simulink model "full_3omni_ctrl_sim_and_exp_with_xpctarget"  (R2014b)
settings: Solver=ode3  SolverMode=SingleTasking  StartTime=0.0  StopTime=40  FixedStep=0.01  RelTol=1e-3
libraries: xpcobsoletelib x13, simulink x10, xpcutilitieslib x3, slrtlib x3
(part 1 of 2)
settings Model: SimulationMode=external  CovMetricSettings=dwe  CovHtmlReporting=off  covSaveCumulativeToWorkspaceVar=off  CovSaveSingleToWorkspaceVar=off  CovExternalEMLEnable=on  CovSFcnEnable=on  Creator=Sarot PC  LastModifiedBy=Sarot PC
settings DataIOCC: LimitDataPoints=off  SaveFormat=StructureWithTime  ReturnWorkspaceOutputs=on
settings OptimizationCC: BlockReduction=off  OptimizeBlockIOStorage=off  BufferReuse=off  GlobalBufferReuse=off  ExpressionFolding=off  LocalBlockOutputs=off
settings DebuggingCC: SolverPrmCheckMsg=none  FrameProcessingCompatibilityMsg=error  SFUnexpectedBacktrackingDiag=error  SFNoUnconditionalDefaultTransitionDiag=error
settings HardwareCC: ProdIntDivRoundTo=Zero  ProdEndianess=LittleEndian  ProdLongLongMode=on  ProdHWDeviceType=Generic->32-bit x86 compatible
settings ModelReferenceCC: PropagateSignalLabelsOutOfModel=on
settings SFSimCC: SimUseLocalCustomCode=on
settings RTWCC: Description=Simulink Real-Time  SystemTargetFile=slrt.tlc  TemplateMakefile=slrt_default_tmf  RTWUseLocalCustomCode=on  CodeExecutionProfiling=on  RTWCompilerOptimization=On
settings SimulinkRealTimeCC: GeneratePreprocessorConditionals=Disable all

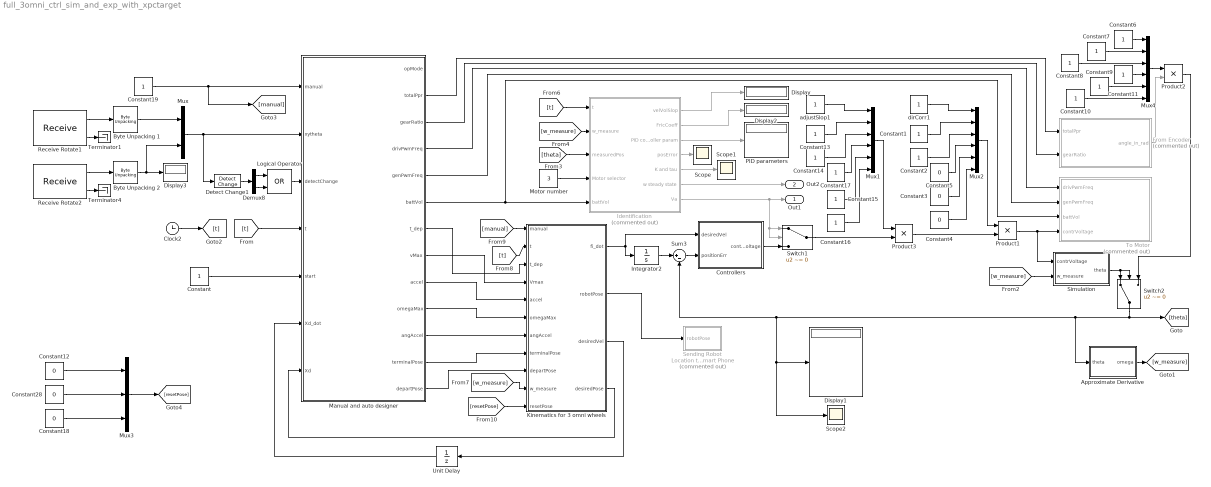
== system full_3omni_ctrl_sim_and_exp_with_xpctarget ==
  Approximate Derivative : Subsystem
  Byte Unpacking 1 : xpcutilitieslib/Byte Unpacking   MaskUnpackedDataTypes={'double'}  MaskUnpackedDataSizes={[1]}  MaskAlignment=1
  Byte Unpacking 2 : xpcutilitieslib/Byte Unpacking   MaskUnpackedDataTypes={'double'}  MaskUnpackedDataSizes={[1]}  MaskAlignment=1
  Clock2 : Clock
  Constant{,1..2,6..11,13..17,19} (15 alike) : Constant
  Constant{3..5,12,18,28} (6 alike) : Constant  Value=0
  Controllers : Subsystem
  Demux8 : Demux  Outputs=2
  Detect Change1 : simulink/Logic and Bit Operations/Detect Change  vinit=0  OutDataTypeStr=boolean
  Display{,1..3} (4 alike) : Display
  From Encoder : Subsystem  Commented=on
  Identification : Subsystem  Commented=on
  Integrator2 : Integrator  InitialCondition=zeros(6,1)
  Kinematics for 3 omni wheels : Subsystem
  Logical Operator : Logic  Operator=OR  AllPortsSameDT=off  OutDataTypeStr=boolean
  Manual and auto designer : Stateflow chart  TreatAsAtomicUnit=on
      settings: PermitHierarchicalResolution=ParametersOnly
  Motor number : Constant  Value=3
  Mux : Mux  Inputs=2
  Mux1 : Mux  Inputs=6
  Mux2 : Mux  Inputs=6
  Mux3 : Mux  Inputs=3
  Mux4 : Mux  Inputs=6
  PID parameters : Display
  Product1 : Product
  Product2 : Product
  Product3 : Product
  Receive Rotate1 : slrtlib/UDP/Receive   ipPort=2501  width=8  ipAddress=192.168.88.233  sampletime=-1
  Receive Rotate2 : slrtlib/UDP/Receive   ipPort=2502  width=8  ipAddress=192.168.88.233  sampletime=-1
  Scope : Scope
      settings: TimeRange=auto  LimitDataPoints=on  MaxDataPoints=3300  SaveToWorkspace=off  SaveName=ScopeData2  YMin=-0.015  YMax=0.015  SampleTime=-1
  Scope1 : Scope
      settings: TimeRange=auto  MaxDataPoints=5000  SaveToWorkspace=off  SaveName=ScopeData3  YMin=-1156.64589  YMax=375.14901  SampleTime=-1
  Scope2 : Scope
      settings: TimeRange=auto  ShowLegends=on  MaxDataPoints=5000  SaveToWorkspace=off  SaveName=ScopeData4  YMin=-1092.82941  YMax=1092.82933  SampleTime=-1
  Sending Robot Location to Smart Phone : Subsystem  Commented=on
  Simulation : Subsystem
  Sum3 : Sum  Inputs=|+-
  Switch1 : Switch  Criteria=u2 ~= 0
  Switch2 : Switch  Criteria=u2 ~= 0
  Terminator1 : Terminator
  Terminator4 : Terminator
  To Motor : Subsystem  Commented=on
  Unit Delay : UnitDelay  InitialCondition=[0;0;0]  SampleTime=-1  HasFrameUpgradeWarning=on
  adjustSlop1 : Constant
  dirCorr1 : Constant
  Out1 : Outport
  Out2 : Outport  Port=2
  wires:
  Constant2/1 -> Mux2/3
  dirCorr1/1 -> Mux2/1
  Constant1/1 -> Mux2/2
  Mux2/1 -> Product1/1
  Product1/1 -> Simulation/1(contrVoltage), To Motor/4(contrVoltage)
  Product3/1 -> Product1/2
  Constant5/1 -> Mux2/4
  Constant3/1 -> Mux2/5
  Constant4/1 -> Mux2/6
  Constant10/1 -> Mux4/6
  Constant6/1 -> Mux4/1
  Constant7/1 -> Mux4/2
  Mux4/1 -> Product2/1
  Constant11/1 -> Mux4/4
  Constant9/1 -> Mux4/5
  Constant8/1 -> Mux4/3
  From Encoder/1(angle_in_rad) -> Product2/2
  Product2/1 -> Switch2/3
  Constant16/1 -> Mux1/6
  Constant15/1 -> Mux1/5
  Constant17/1 -> Mux1/4
  Mux1/1 -> Product3/1
  Constant13/1 -> Mux1/2
  adjustSlop1/1 -> Mux1/1
  Constant14/1 -> Mux1/3
  Switch1/1 -> Product3/2
  Manual and auto designer/2(totalPpr) -> From Encoder/1(totalPpr)
  Manual and auto designer/3(gearRatio) -> From Encoder/2(gearRatio)
  Simulation/1(theta) -> Switch2/2, Switch2/1
  Approximate Derivative/1(omega) -> [w_measure]
  Controllers/1(contrVoltage) -> Switch1/3
  Sum3/1 -> Controllers/2(positionErr)
  Identification/7(Va) -> Out1/1, Switch1/2, Switch1/1
  [t] -> Identification/1(t)
  [w_measure] -> Identification/2(w_measure)
  [theta] -> Identification/3(measuredPos)
  Identification/1(velVolSlop) -> Display/1
  Identification/3(PID controller param) -> PID parameters/1
  Identification/6(w steady state) -> Out2/1
  Identification/4(posError) -> Scope/1
  Identification/5(K and tau) -> Scope1/1
  Motor number/1 -> Identification/4(Motor selector)
  Integrator2/1 -> Sum3/1
  Kinematics for 3 omni wheels/1(fi_dot) -> Integrator2/1, Controllers/1(desiredVel)
  Switch2/1 -> Approximate Derivative/1(theta), Sum3/2, Scope2/1, Display1/1, [theta]
  Manual and auto designer/4(drivPwmFreq) -> To Motor/1(drivPwmFreq)
  Manual and auto designer/5(genPwmFreq) -> To Motor/2(genPwmFreq)
  Manual and auto designer/6(battVol) -> To Motor/3(battVol), Identification/5(battVol)
  Identification/2(FricCoeff) -> Display2/1
  [w_measure] -> Simulation/2(w_measure)
  Demux8/2 -> Logical Operator/2
  Logical Operator/1 -> Manual and auto designer/3(detectChange)
  Mux/1 -> Detect Change1/1, Manual and auto designer/2(xytheta)
  Detect Change1/1 -> Demux8/1
  Kinematics for 3 omni wheels/4(desiredPose) -> Manual and auto designer/7(Xd)
  [t] -> Manual and auto designer/4(t)
  Constant/1 -> Manual and auto designer/5(start)
  Demux8/1 -> Logical Operator/1
  Constant19/1 -> [manual], Manual and auto designer/1(manual)
  Clock2/1 -> [t]
  [t] -> Kinematics for 3 omni wheels/2(t)
  Kinematics for 3 omni wheels/2(robotPose) -> Sending Robot Location to Smart Phone/1(robotPose)
  [w_measure] -> Kinematics for 3 omni wheels/10(w_measure)
  Kinematics for 3 omni wheels/3(desiredVel) -> Unit Delay/1
  Manual and auto designer/13(departPose) -> Kinematics for 3 omni wheels/9(departPose)
  Manual and auto designer/12(terminalPose) -> Kinematics for 3 omni wheels/8(terminalPose)
  Manual and auto designer/10(omegaMax) -> Kinematics for 3 omni wheels/6(omegaMax)
  Manual and auto designer/11(angAccel) -> Kinematics for 3 omni wheels/7(angAccel)
  Manual and auto designer/9(accel) -> Kinematics for 3 omni wheels/5(accel)
  Manual and auto designer/8(vMax) -> Kinematics for 3 omni wheels/4(Vmax)
  Manual and auto designer/7(t_dep) -> Kinematics for 3 omni wheels/3(t_dep)
  [manual] -> Kinematics for 3 omni wheels/1(manual)
  Unit Delay/1 -> Manual and auto designer/6(Xd_dot)
  Constant12/1 -> Mux3/1
  Constant28/1 -> Mux3/2
  Constant18/1 -> Mux3/3
  Mux3/1 -> [resetPose]
  [resetPose] -> Kinematics for 3 omni wheels/11(resetPose)
  Receive Rotate2/1 -> Byte Unpacking 2/1
  Receive Rotate1/2 -> Terminator1/1
  Byte Unpacking 1/1 -> Mux/1
  Receive Rotate2/2 -> Terminator4/1
  Receive Rotate1/1 -> Byte Unpacking 1/1
  Byte Unpacking 2/1 -> Mux/2, Display3/1

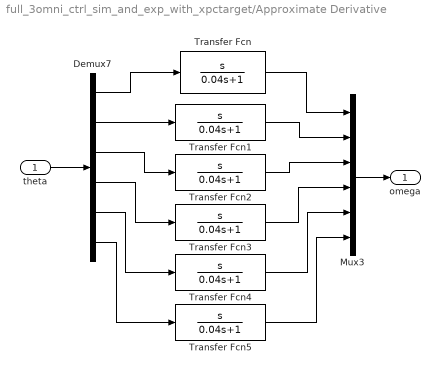
== system full_3omni_ctrl_sim_and_exp_with_xpctarget/Approximate Derivative ==
  theta : Inport
  Demux7 : Demux  Outputs=6
  Mux3 : Mux  Inputs=6
  Transfer Fcn{,1..5} (6 alike) : TransferFcn  Numerator=[1 0]  Denominator=[0.04 1]
  omega : Outport
  wires:
  Transfer Fcn1/1 -> Mux3/2
  Demux7/5 -> Transfer Fcn4/1
  Transfer Fcn3/1 -> Mux3/4
  Demux7/3 -> Transfer Fcn2/1
  Demux7/6 -> Transfer Fcn5/1
  Transfer Fcn2/1 -> Mux3/3
  Transfer Fcn/1 -> Mux3/1
  Transfer Fcn5/1 -> Mux3/6
  Demux7/4 -> Transfer Fcn3/1
  Mux3/1 -> omega/1
  Transfer Fcn4/1 -> Mux3/5
  Demux7/1 -> Transfer Fcn/1
  Demux7/2 -> Transfer Fcn1/1
  theta/1 -> Demux7/1

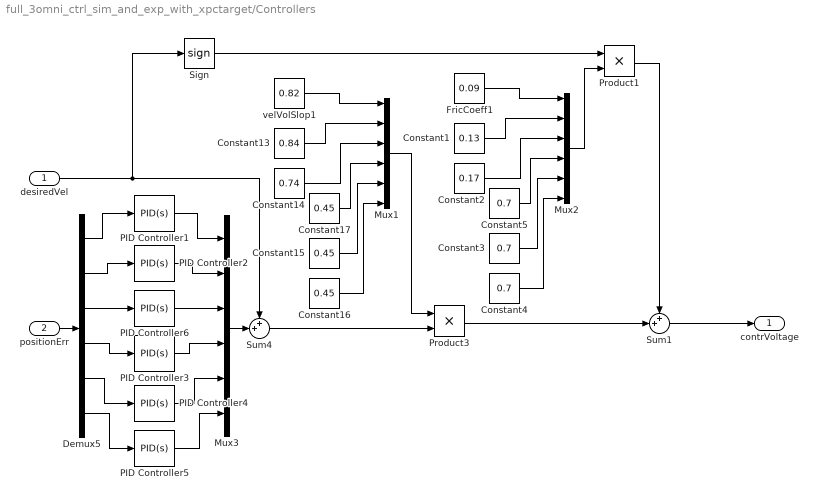
== system full_3omni_ctrl_sim_and_exp_with_xpctarget/Controllers ==
  desiredVel : Inport
  positionErr : Inport  Port=2
  Constant1 : Constant  Value=0.13
  Constant13 : Constant  Value=0.84
  Constant14 : Constant  Value=0.74
  Constant15 : Constant  Value=0.45
  Constant16 : Constant  Value=0.45
  Constant17 : Constant  Value=0.45
  Constant2 : Constant  Value=0.17
  Constant3 : Constant  Value=0.7
  Constant4 : Constant  Value=0.7
  Constant5 : Constant  Value=0.7
  Demux5 : Demux  Outputs=6
  FricCoeff1 : Constant  Value=0.09
  Mux1 : Mux  Inputs=6
  Mux2 : Mux  Inputs=6
  Mux3 : Mux  Inputs=6
  "PID Controller1 " : simulink/Continuous/PID Controller  Controller=PID  Form=Parallel  TimeDomain=Continuous-time  SampleTime=-1  IntegratorMethod=Forward Euler  FilterMethod=Forward Euler  ControllerParametersSource=internal  P=45/0.82  I=0  D=2.9/0.82  UseFilter=on  N=100  InitialConditionSource=internal  InitialConditionForIntegrator=0  InitialConditionForFilter=0  DifferentiatorICPrevScaledInput=0  ExternalReset=none  TrackingMode=off  Kt=1  LimitOutput=off  UpperSaturationLimit=inf  LowerSaturationLimit=-inf  LinearizeAsGain=on  AntiWindupMode=none  Kb=1  POutMin=[]  POutMax=[]  IOutMin=[]  IOutMax=[]  DOutMin=[]  DOutMax=[]  NOutMin=[]  NOutMax=[]  SumOutMin=[]  SumOutMax=[]  SaturationOutMin=[]  SaturationOutMax=[]  PParamMin=[]  PParamMax=[]  IParamMin=[]  IParamMax=[]  DParamMin=[]  DParamMax=[]  NParamMin=[]  NParamMax=[]  KbParamMin=[]  KbParamMax=[]  KtParamMin=[]  KtParamMax=[]  KbOutMin=[]  KbOutMax=[]  KtOutMin=[]  KtOutMax=[]  IntegratorOutMin=[]  IntegratorOutMax=[]  FilterOutMin=[]  FilterOutMax=[]  SumI1OutMin=[]  SumI1OutMax=[]  SumI2OutMin=[]  SumI2OutMax=[]  SumI3OutMin=[]  SumI3OutMax=[]  SumDOutMin=[]  SumDOutMax=[]  DifferentiatorOutMin=[]  DifferentiatorOutMax=[]  IntegratorContinuousStateAttributes=''  IntegratorStateMustResolveToSignalObject=off  IntegratorRTWStateStorageClass=Auto  FilterContinuousStateAttributes=''  FilterStateMustResolveToSignalObject=off  FilterRTWStateStorageClass=Auto
  PID Controller2 : simulink/Continuous/PID Controller  Controller=PID  Form=Parallel  TimeDomain=Continuous-time  SampleTime=-1  IntegratorMethod=Forward Euler  FilterMethod=Forward Euler  ControllerParametersSource=internal  P=45/0.84  I=0  D=2.96/0.84  UseFilter=on  N=100  InitialConditionSource=internal  InitialConditionForIntegrator=0  InitialConditionForFilter=0  DifferentiatorICPrevScaledInput=0  ExternalReset=none  TrackingMode=off  Kt=1  LimitOutput=off  UpperSaturationLimit=inf  LowerSaturationLimit=-inf  LinearizeAsGain=on  AntiWindupMode=none  Kb=1  POutMin=[]  POutMax=[]  IOutMin=[]  IOutMax=[]  DOutMin=[]  DOutMax=[]  NOutMin=[]  NOutMax=[]  SumOutMin=[]  SumOutMax=[]  SaturationOutMin=[]  SaturationOutMax=[]  PParamMin=[]  PParamMax=[]  IParamMin=[]  IParamMax=[]  DParamMin=[]  DParamMax=[]  NParamMin=[]  NParamMax=[]  KbParamMin=[]  KbParamMax=[]  KtParamMin=[]  KtParamMax=[]  KbOutMin=[]  KbOutMax=[]  KtOutMin=[]  KtOutMax=[]  IntegratorOutMin=[]  IntegratorOutMax=[]  FilterOutMin=[]  FilterOutMax=[]  SumI1OutMin=[]  SumI1OutMax=[]  SumI2OutMin=[]  SumI2OutMax=[]  SumI3OutMin=[]  SumI3OutMax=[]  SumDOutMin=[]  SumDOutMax=[]  DifferentiatorOutMin=[]  DifferentiatorOutMax=[]  IntegratorContinuousStateAttributes=''  IntegratorStateMustResolveToSignalObject=off  IntegratorRTWStateStorageClass=Auto  FilterContinuousStateAttributes=''  FilterStateMustResolveToSignalObject=off  FilterRTWStateStorageClass=Auto
  PID Controller3 : simulink/Continuous/PID Controller  Controller=PID  Form=Parallel  TimeDomain=Continuous-time  SampleTime=-1  IntegratorMethod=Forward Euler  FilterMethod=Forward Euler  ControllerParametersSource=internal  P=10  I=0  D=3  UseFilter=on  N=100  InitialConditionSource=internal  InitialConditionForIntegrator=0  InitialConditionForFilter=0  DifferentiatorICPrevScaledInput=0  ExternalReset=none  TrackingMode=off  Kt=1  LimitOutput=off  UpperSaturationLimit=inf  LowerSaturationLimit=-inf  LinearizeAsGain=on  AntiWindupMode=none  Kb=1  POutMin=[]  POutMax=[]  IOutMin=[]  IOutMax=[]  DOutMin=[]  DOutMax=[]  NOutMin=[]  NOutMax=[]  SumOutMin=[]  SumOutMax=[]  SaturationOutMin=[]  SaturationOutMax=[]  PParamMin=[]  PParamMax=[]  IParamMin=[]  IParamMax=[]  DParamMin=[]  DParamMax=[]  NParamMin=[]  NParamMax=[]  KbParamMin=[]  KbParamMax=[]  KtParamMin=[]  KtParamMax=[]  KbOutMin=[]  KbOutMax=[]  KtOutMin=[]  KtOutMax=[]  IntegratorOutMin=[]  IntegratorOutMax=[]  FilterOutMin=[]  FilterOutMax=[]  SumI1OutMin=[]  SumI1OutMax=[]  SumI2OutMin=[]  SumI2OutMax=[]  SumI3OutMin=[]  SumI3OutMax=[]  SumDOutMin=[]  SumDOutMax=[]  DifferentiatorOutMin=[]  DifferentiatorOutMax=[]  IntegratorContinuousStateAttributes=''  IntegratorStateMustResolveToSignalObject=off  IntegratorRTWStateStorageClass=Auto  FilterContinuousStateAttributes=''  FilterStateMustResolveToSignalObject=off  FilterRTWStateStorageClass=Auto
  PID Controller4 : simulink/Continuous/PID Controller  Controller=PID  Form=Parallel  TimeDomain=Continuous-time  SampleTime=-1  IntegratorMethod=Forward Euler  FilterMethod=Forward Euler  ControllerParametersSource=internal  P=10  I=0  D=3  UseFilter=on  N=100  InitialConditionSource=internal  InitialConditionForIntegrator=0  InitialConditionForFilter=0  DifferentiatorICPrevScaledInput=0  ExternalReset=none  TrackingMode=off  Kt=1  LimitOutput=off  UpperSaturationLimit=inf  LowerSaturationLimit=-inf  LinearizeAsGain=on  AntiWindupMode=none  Kb=1  POutMin=[]  POutMax=[]  IOutMin=[]  IOutMax=[]  DOutMin=[]  DOutMax=[]  NOutMin=[]  NOutMax=[]  SumOutMin=[]  SumOutMax=[]  SaturationOutMin=[]  SaturationOutMax=[]  PParamMin=[]  PParamMax=[]  IParamMin=[]  IParamMax=[]  DParamMin=[]  DParamMax=[]  NParamMin=[]  NParamMax=[]  KbParamMin=[]  KbParamMax=[]  KtParamMin=[]  KtParamMax=[]  KbOutMin=[]  KbOutMax=[]  KtOutMin=[]  KtOutMax=[]  IntegratorOutMin=[]  IntegratorOutMax=[]  FilterOutMin=[]  FilterOutMax=[]  SumI1OutMin=[]  SumI1OutMax=[]  SumI2OutMin=[]  SumI2OutMax=[]  SumI3OutMin=[]  SumI3OutMax=[]  SumDOutMin=[]  SumDOutMax=[]  DifferentiatorOutMin=[]  DifferentiatorOutMax=[]  IntegratorContinuousStateAttributes=''  IntegratorStateMustResolveToSignalObject=off  IntegratorRTWStateStorageClass=Auto  FilterContinuousStateAttributes=''  FilterStateMustResolveToSignalObject=off  FilterRTWStateStorageClass=Auto
  PID Controller5 : simulink/Continuous/PID Controller  Controller=PID  Form=Parallel  TimeDomain=Continuous-time  SampleTime=-1  IntegratorMethod=Forward Euler  FilterMethod=Forward Euler  ControllerParametersSource=internal  P=10  I=0  D=3  UseFilter=on  N=100  InitialConditionSource=internal  InitialConditionForIntegrator=0  InitialConditionForFilter=0  DifferentiatorICPrevScaledInput=0  ExternalReset=none  TrackingMode=off  Kt=1  LimitOutput=off  UpperSaturationLimit=inf  LowerSaturationLimit=-inf  LinearizeAsGain=on  AntiWindupMode=none  Kb=1  POutMin=[]  POutMax=[]  IOutMin=[]  IOutMax=[]  DOutMin=[]  DOutMax=[]  NOutMin=[]  NOutMax=[]  SumOutMin=[]  SumOutMax=[]  SaturationOutMin=[]  SaturationOutMax=[]  PParamMin=[]  PParamMax=[]  IParamMin=[]  IParamMax=[]  DParamMin=[]  DParamMax=[]  NParamMin=[]  NParamMax=[]  KbParamMin=[]  KbParamMax=[]  KtParamMin=[]  KtParamMax=[]  KbOutMin=[]  KbOutMax=[]  KtOutMin=[]  KtOutMax=[]  IntegratorOutMin=[]  IntegratorOutMax=[]  FilterOutMin=[]  FilterOutMax=[]  SumI1OutMin=[]  SumI1OutMax=[]  SumI2OutMin=[]  SumI2OutMax=[]  SumI3OutMin=[]  SumI3OutMax=[]  SumDOutMin=[]  SumDOutMax=[]  DifferentiatorOutMin=[]  DifferentiatorOutMax=[]  IntegratorContinuousStateAttributes=''  IntegratorStateMustResolveToSignalObject=off  IntegratorRTWStateStorageClass=Auto  FilterContinuousStateAttributes=''  FilterStateMustResolveToSignalObject=off  FilterRTWStateStorageClass=Auto
  PID Controller6 : simulink/Continuous/PID Controller  Controller=PID  Form=Parallel  TimeDomain=Continuous-time  SampleTime=-1  IntegratorMethod=Forward Euler  FilterMethod=Forward Euler  ControllerParametersSource=internal  P=45/0.74  I=0  D=2.59/0.74  UseFilter=on  N=100  InitialConditionSource=internal  InitialConditionForIntegrator=0  InitialConditionForFilter=0  DifferentiatorICPrevScaledInput=0  ExternalReset=none  TrackingMode=off  Kt=1  LimitOutput=off  UpperSaturationLimit=inf  LowerSaturationLimit=-inf  LinearizeAsGain=on  AntiWindupMode=none  Kb=1  POutMin=[]  POutMax=[]  IOutMin=[]  IOutMax=[]  DOutMin=[]  DOutMax=[]  NOutMin=[]  NOutMax=[]  SumOutMin=[]  SumOutMax=[]  SaturationOutMin=[]  SaturationOutMax=[]  PParamMin=[]  PParamMax=[]  IParamMin=[]  IParamMax=[]  DParamMin=[]  DParamMax=[]  NParamMin=[]  NParamMax=[]  KbParamMin=[]  KbParamMax=[]  KtParamMin=[]  KtParamMax=[]  KbOutMin=[]  KbOutMax=[]  KtOutMin=[]  KtOutMax=[]  IntegratorOutMin=[]  IntegratorOutMax=[]  FilterOutMin=[]  FilterOutMax=[]  SumI1OutMin=[]  SumI1OutMax=[]  SumI2OutMin=[]  SumI2OutMax=[]  SumI3OutMin=[]  SumI3OutMax=[]  SumDOutMin=[]  SumDOutMax=[]  DifferentiatorOutMin=[]  DifferentiatorOutMax=[]  IntegratorContinuousStateAttributes=''  IntegratorStateMustResolveToSignalObject=off  IntegratorRTWStateStorageClass=Auto  FilterContinuousStateAttributes=''  FilterStateMustResolveToSignalObject=off  FilterRTWStateStorageClass=Auto
  Product1 : Product
  Product3 : Product
  Sign : Signum
  Sum1 : Sum  Inputs=++|
  Sum4 : Sum  Inputs=++|
  velVolSlop1 : Constant  Value=0.82
  contrVoltage : Outport
  wires:
  PID Controller2/1 -> Mux3/2
  Demux5/3 -> PID Controller6/1
  Demux5/1 -> "PID Controller1 "/1
  PID Controller6/1 -> Mux3/3
  "PID Controller1 "/1 -> Mux3/1
  positionErr/1 -> Demux5/1
  Demux5/2 -> PID Controller2/1
  Demux5/4 -> PID Controller3/1
  Demux5/5 -> PID Controller4/1
  Demux5/6 -> PID Controller5/1
  PID Controller3/1 -> Mux3/4
  PID Controller4/1 -> Mux3/5
  PID Controller5/1 -> Mux3/6
  Constant16/1 -> Mux1/6
  Constant15/1 -> Mux1/5
  Constant14/1 -> Mux1/3
  Constant13/1 -> Mux1/2
  velVolSlop1/1 -> Mux1/1
  Mux1/1 -> Product3/1
  Constant17/1 -> Mux1/4
  Sum1/1 -> contrVoltage/1
  Mux3/1 -> Sum4/2
  Sum4/1 -> Product3/2
  desiredVel/1 -> Sign/1, Sum4/1
  Product3/1 -> Sum1/2
  Constant2/1 -> Mux2/3
  Constant5/1 -> Mux2/4
  FricCoeff1/1 -> Mux2/1
  Constant4/1 -> Mux2/6
  Constant3/1 -> Mux2/5
  Constant1/1 -> Mux2/2
  Sign/1 -> Product1/1
  Mux2/1 -> Product1/2
  Product1/1 -> Sum1/1

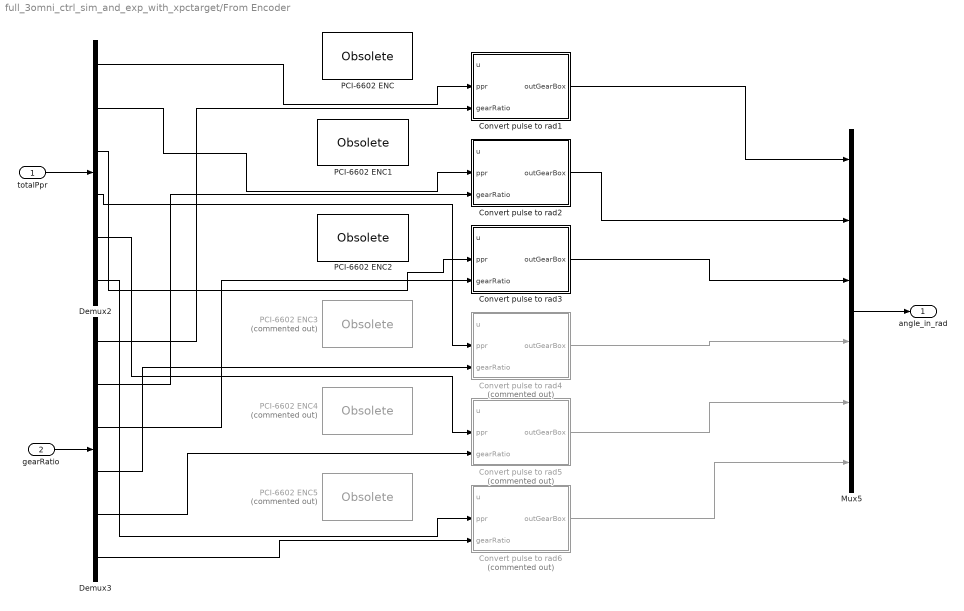
== system full_3omni_ctrl_sim_and_exp_with_xpctarget/From Encoder ==
  totalPpr : Inport
  gearRatio : Inport  Port=2
  Convert pulse to rad1 : MATLAB Function  TreatAsAtomicUnit=on
      settings: PermitHierarchicalResolution=ParametersOnly
  Convert pulse to rad2 : MATLAB Function  TreatAsAtomicUnit=on
      settings: PermitHierarchicalResolution=ParametersOnly
  Convert pulse to rad3 : MATLAB Function  TreatAsAtomicUnit=on
      settings: PermitHierarchicalResolution=ParametersOnly
  Convert pulse to rad4 : MATLAB Function  Commented=on  TreatAsAtomicUnit=on
      settings: PermitHierarchicalResolution=ParametersOnly
  Convert pulse to rad5 : MATLAB Function  Commented=on  TreatAsAtomicUnit=on
      settings: PermitHierarchicalResolution=ParametersOnly
  Convert pulse to rad6 : MATLAB Function  Commented=on  TreatAsAtomicUnit=on
      settings: PermitHierarchicalResolution=ParametersOnly
  Demux2 : Demux  Outputs=6
  Demux3 : Demux  Outputs=6
  Mux5 : Mux  Inputs=6
  PCI-6602 ENC : xpcobsoletelib/Obsolete
  PCI-6602 ENC1 : xpcobsoletelib/Obsolete
  PCI-6602 ENC2 : xpcobsoletelib/Obsolete
  PCI-6602 ENC3 : xpcobsoletelib/Obsolete  Commented=on
  PCI-6602 ENC4 : xpcobsoletelib/Obsolete  Commented=on
  PCI-6602 ENC5 : xpcobsoletelib/Obsolete  Commented=on
  angle_in_rad : Outport
  wires:
  Demux3/5 -> Convert pulse to rad5/3(gearRatio)
  Demux3/6 -> Convert pulse to rad6/3(gearRatio)
  Demux3/1 -> Convert pulse to rad1/3(gearRatio)
  Convert pulse to rad3/1(outGearBox) -> Mux5/3
  Convert pulse to rad5/1(outGearBox) -> Mux5/5
  Mux5/1 -> angle_in_rad/1
  Demux2/2 -> Convert pulse to rad2/2(ppr)
  gearRatio/1 -> Demux3/1
  ? -> Convert pulse to rad5/1(u)
  Demux2/5 -> Convert pulse to rad5/2(ppr)
  ? -> Convert pulse to rad4/1(u)
  Demux2/6 -> Convert pulse to rad6/2(ppr)
  Demux2/3 -> Convert pulse to rad3/2(ppr)
  Demux3/3 -> Convert pulse to rad3/3(gearRatio)
  ? -> Convert pulse to rad2/1(u)
  Demux2/4 -> Convert pulse to rad4/2(ppr)
  Demux2/1 -> Convert pulse to rad1/2(ppr)
  Convert pulse to rad6/1(outGearBox) -> Mux5/6
  Demux3/4 -> Convert pulse to rad4/3(gearRatio)
  Convert pulse to rad1/1(outGearBox) -> Mux5/1
  ? -> Convert pulse to rad3/1(u)
  Convert pulse to rad4/1(outGearBox) -> Mux5/4
  Demux3/2 -> Convert pulse to rad2/3(gearRatio)
  Convert pulse to rad2/1(outGearBox) -> Mux5/2
  totalPpr/1 -> Demux2/1
  ? -> Convert pulse to rad6/1(u)
  ? -> Convert pulse to rad1/1(u)

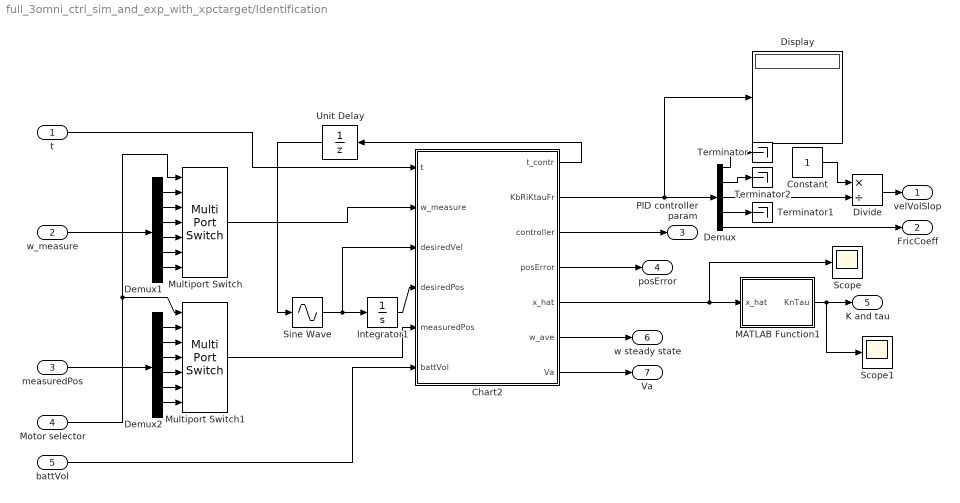
== system full_3omni_ctrl_sim_and_exp_with_xpctarget/Identification ==
  t : Inport
  w_measure : Inport  Port=2
  measuredPos : Inport  Port=3
  Motor selector : Inport  Port=4
  battVol : Inport  Port=5
  Chart2 : Stateflow chart  TreatAsAtomicUnit=on
      settings: PermitHierarchicalResolution=ParametersOnly
  Constant : Constant
  Demux : Demux  Outputs=5
  Demux1 : Demux  Outputs=6
  Demux2 : Demux  Outputs=6
  Display : Display
  Divide : Product  Inputs=*/
  Integrator1 : Integrator
  MATLAB Function1 : MATLAB Function  TreatAsAtomicUnit=on
      settings: PermitHierarchicalResolution=ParametersOnly
  Multiport Switch : MultiPortSwitch  Inputs=6
  Multiport Switch1 : MultiPortSwitch  Inputs=6
  Scope : Scope
      settings: TimeRange=auto  ShowLegends=on  LimitDataPoints=on  MaxDataPoints=50000  SaveToWorkspace=off  SaveName=ScopeData  YMin=-20  YMax=20  SampleTime=-1
  Scope1 : Scope
      settings: TimeRange=auto  LimitDataPoints=on  MaxDataPoints=50000  SaveToWorkspace=off  YMin=-188.99586  YMax=585.89399  SampleTime=-1
  Sine Wave : Sin  TimeSource=Use external signal  Amplitude=pi  SampleTime=0
  Terminator : Terminator
  Terminator1 : Terminator
  Terminator2 : Terminator
  Unit Delay : UnitDelay  SampleTime=-1  HasFrameUpgradeWarning=on
  velVolSlop : Outport
  FricCoeff : Outport  Port=2
  PID controller param : Outport  Port=3
  posError : Outport  Port=4
  K and tau : Outport  Port=5
  w steady state : Outport  Port=6
  Va : Outport  Port=7
  wires:
  Sine Wave/1 -> Chart2/3(desiredVel), Integrator1/1
  Chart2/5(x_hat) -> Scope/1, MATLAB Function1/1(x_hat)
  Multiport Switch/1 -> Chart2/2(w_measure)
  Chart2/7(Va) -> Va/1
  Chart2/1(t_contr) -> Unit Delay/1
  Integrator1/1 -> Chart2/4(desiredPos)
  Unit Delay/1 -> Sine Wave/1
  Chart2/4(posError) -> posError/1
  MATLAB Function1/1(KnTau) -> Scope1/1, K and tau/1
  Multiport Switch1/1 -> Chart2/5(measuredPos)
  t/1 -> Chart2/1(t)
  Chart2/2(KbRiKtauFr) -> Display/1, Demux/1
  Chart2/3(controller) -> PID controller param/1
  Chart2/6(w_ave) -> w steady state/1
  Demux/3 -> Divide/2
  Divide/1 -> velVolSlop/1
  Constant/1 -> Divide/1
  Demux/1 -> Terminator/1
  Demux/4 -> Terminator1/1
  Demux/2 -> Terminator2/1
  Demux1/1 -> Multiport Switch/2
  Demux1/2 -> Multiport Switch/3
  Demux1/3 -> Multiport Switch/4
  Demux1/4 -> Multiport Switch/5
  Demux1/5 -> Multiport Switch/6
  Demux1/6 -> Multiport Switch/7
  Demux2/1 -> Multiport Switch1/2
  Demux2/2 -> Multiport Switch1/3
  Demux2/3 -> Multiport Switch1/4
  Demux2/4 -> Multiport Switch1/5
  Demux2/5 -> Multiport Switch1/6
  Demux2/6 -> Multiport Switch1/7
  measuredPos/1 -> Demux2/1
  w_measure/1 -> Demux1/1
  Motor selector/1 -> Multiport Switch1/1, Multiport Switch/1
  Demux/5 -> FricCoeff/1
  battVol/1 -> Chart2/6(battVol)

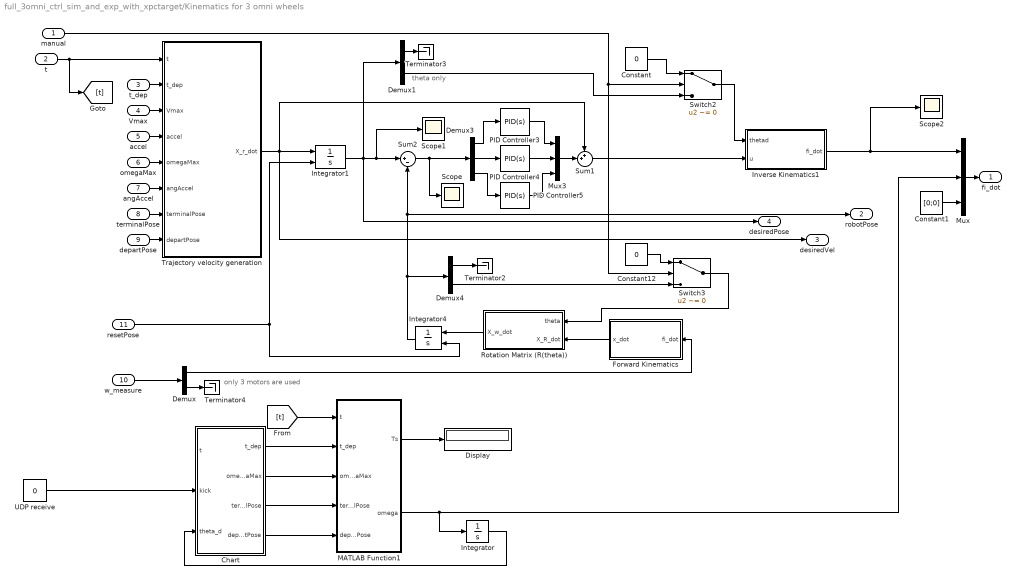
== system full_3omni_ctrl_sim_and_exp_with_xpctarget/Kinematics for 3 omni wheels ==
  note: only 3 motors are used
  note: theta only
  manual : Inport
  t : Inport  Port=2
  t_dep : Inport  Port=3
  Vmax : Inport  Port=4
  accel : Inport  Port=5
  omegaMax : Inport  Port=6
  angAccel : Inport  Port=7
  terminalPose : Inport  Port=8
  departPose : Inport  Port=9
  w_measure : Inport  Port=10
  resetPose : Inport  Port=11
  Chart : Stateflow chart  TreatAsAtomicUnit=on
      settings: PermitHierarchicalResolution=ParametersOnly
  Constant : Constant  Value=0
  Constant1 : Constant  Value=[0;0]
  Constant12 : Constant  Value=0
  Demux : Demux  Outputs=[3,3]
  Demux1 : Demux  Outputs=[2,1]
  Demux3 : Demux  Outputs=3
  Demux4 : Demux  Outputs=[2,1]
  Display : Display
  Forward Kinematics : MATLAB Function  TreatAsAtomicUnit=on
      settings: PermitHierarchicalResolution=ParametersOnly
  Integrator : Integrator
  Integrator1 : Integrator  ExternalReset=either  InitialCondition=[0;0;0]
  Integrator4 : Integrator  ExternalReset=either  InitialCondition=[0;0;0]
  Inverse Kinematics1 : MATLAB Function  TreatAsAtomicUnit=on
      settings: PermitHierarchicalResolution=ParametersOnly
  MATLAB Function1 : MATLAB Function  TreatAsAtomicUnit=on
      settings: PermitHierarchicalResolution=ParametersOnly
  Mux : Mux  Inputs=[3,1,2]
  Mux3 : Mux  Inputs=3
  PID Controller3 : simulink/Continuous/PID Controller  Controller=PID  Form=Parallel  TimeDomain=Continuous-time  SampleTime=-1  IntegratorMethod=Forward Euler  FilterMethod=Forward Euler  ControllerParametersSource=internal  P=5  I=5  D=0  UseFilter=on  N=100  InitialConditionSource=internal  InitialConditionForIntegrator=0  InitialConditionForFilter=0  DifferentiatorICPrevScaledInput=0  ExternalReset=none  TrackingMode=off  Kt=1  LimitOutput=off  UpperSaturationLimit=inf  LowerSaturationLimit=-inf  LinearizeAsGain=on  AntiWindupMode=none  Kb=1  POutMin=[]  POutMax=[]  IOutMin=[]  IOutMax=[]  DOutMin=[]  DOutMax=[]  NOutMin=[]  NOutMax=[]  SumOutMin=[]  SumOutMax=[]  SaturationOutMin=[]  SaturationOutMax=[]  PParamMin=[]  PParamMax=[]  IParamMin=[]  IParamMax=[]  DParamMin=[]  DParamMax=[]  NParamMin=[]  NParamMax=[]  KbParamMin=[]  KbParamMax=[]  KtParamMin=[]  KtParamMax=[]  KbOutMin=[]  KbOutMax=[]  KtOutMin=[]  KtOutMax=[]  IntegratorOutMin=[]  IntegratorOutMax=[]  FilterOutMin=[]  FilterOutMax=[]  SumI1OutMin=[]  SumI1OutMax=[]  SumI2OutMin=[]  SumI2OutMax=[]  SumI3OutMin=[]  SumI3OutMax=[]  SumDOutMin=[]  SumDOutMax=[]  DifferentiatorOutMin=[]  DifferentiatorOutMax=[]  IntegratorContinuousStateAttributes=''  IntegratorStateMustResolveToSignalObject=off  IntegratorRTWStateStorageClass=Auto  FilterContinuousStateAttributes=''  FilterStateMustResolveToSignalObject=off  FilterRTWStateStorageClass=Auto
  PID Controller4 : simulink/Continuous/PID Controller  Controller=PID  Form=Parallel  TimeDomain=Continuous-time  SampleTime=-1  IntegratorMethod=Forward Euler  FilterMethod=Forward Euler  ControllerParametersSource=internal  P=5  I=5  D=0  UseFilter=on  N=100  InitialConditionSource=internal  InitialConditionForIntegrator=0  InitialConditionForFilter=0  DifferentiatorICPrevScaledInput=0  ExternalReset=none  TrackingMode=off  Kt=1  LimitOutput=off  UpperSaturationLimit=inf  LowerSaturationLimit=-inf  LinearizeAsGain=on  AntiWindupMode=none  Kb=1  POutMin=[]  POutMax=[]  IOutMin=[]  IOutMax=[]  DOutMin=[]  DOutMax=[]  NOutMin=[]  NOutMax=[]  SumOutMin=[]  SumOutMax=[]  SaturationOutMin=[]  SaturationOutMax=[]  PParamMin=[]  PParamMax=[]  IParamMin=[]  IParamMax=[]  DParamMin=[]  DParamMax=[]  NParamMin=[]  NParamMax=[]  KbParamMin=[]  KbParamMax=[]  KtParamMin=[]  KtParamMax=[]  KbOutMin=[]  KbOutMax=[]  KtOutMin=[]  KtOutMax=[]  IntegratorOutMin=[]  IntegratorOutMax=[]  FilterOutMin=[]  FilterOutMax=[]  SumI1OutMin=[]  SumI1OutMax=[]  SumI2OutMin=[]  SumI2OutMax=[]  SumI3OutMin=[]  SumI3OutMax=[]  SumDOutMin=[]  SumDOutMax=[]  DifferentiatorOutMin=[]  DifferentiatorOutMax=[]  IntegratorContinuousStateAttributes=''  IntegratorStateMustResolveToSignalObject=off  IntegratorRTWStateStorageClass=Auto  FilterContinuousStateAttributes=''  FilterStateMustResolveToSignalObject=off  FilterRTWStateStorageClass=Auto
  PID Controller5 : simulink/Continuous/PID Controller  Controller=PID  Form=Parallel  TimeDomain=Continuous-time  SampleTime=-1  IntegratorMethod=Forward Euler  FilterMethod=Forward Euler  ControllerParametersSource=internal  P=5  I=5  D=0  UseFilter=on  N=100  InitialConditionSource=internal  InitialConditionForIntegrator=0  InitialConditionForFilter=0  DifferentiatorICPrevScaledInput=0  ExternalReset=none  TrackingMode=off  Kt=1  LimitOutput=off  UpperSaturationLimit=inf  LowerSaturationLimit=-inf  LinearizeAsGain=on  AntiWindupMode=none  Kb=1  POutMin=[]  POutMax=[]  IOutMin=[]  IOutMax=[]  DOutMin=[]  DOutMax=[]  NOutMin=[]  NOutMax=[]  SumOutMin=[]  SumOutMax=[]  SaturationOutMin=[]  SaturationOutMax=[]  PParamMin=[]  PParamMax=[]  IParamMin=[]  IParamMax=[]  DParamMin=[]  DParamMax=[]  NParamMin=[]  NParamMax=[]  KbParamMin=[]  KbParamMax=[]  KtParamMin=[]  KtParamMax=[]  KbOutMin=[]  KbOutMax=[]  KtOutMin=[]  KtOutMax=[]  IntegratorOutMin=[]  IntegratorOutMax=[]  FilterOutMin=[]  FilterOutMax=[]  SumI1OutMin=[]  SumI1OutMax=[]  SumI2OutMin=[]  SumI2OutMax=[]  SumI3OutMin=[]  SumI3OutMax=[]  SumDOutMin=[]  SumDOutMax=[]  DifferentiatorOutMin=[]  DifferentiatorOutMax=[]  IntegratorContinuousStateAttributes=''  IntegratorStateMustResolveToSignalObject=off  IntegratorRTWStateStorageClass=Auto  FilterContinuousStateAttributes=''  FilterStateMustResolveToSignalObject=off  FilterRTWStateStorageClass=Auto
  Rotation Matrix (R(theta)) : MATLAB Function  TreatAsAtomicUnit=on
      settings: PermitHierarchicalResolution=ParametersOnly
  Scope : Scope
      settings: TimeRange=auto  MaxDataPoints=5000  SaveToWorkspace=off  SaveName=ScopeData5  YMin=-0.0293  YMax=0.02321  SampleTime=-1
  Scope1 : Scope
      settings: TimeRange=auto  MaxDataPoints=5000  SaveToWorkspace=off  SaveName=ScopeData6  YMin=-9.4975  YMax=85.47747  SampleTime=-1
  Scope2 : Scope
      settings: TimeRange=auto  MaxDataPoints=5000  SaveToWorkspace=off  SaveName=ScopeData9  YMin=-19395.70683  YMax=19395.73611  SampleTime=-1
  Sum1 : Sum  Inputs=++|
  Sum2 : Sum  Inputs=|+-
  Switch2 : Switch  Criteria=u2 ~= 0
  Switch3 : Switch  Criteria=u2 ~= 0
  Terminator2 : Terminator
  Terminator3 : Terminator
  Terminator4 : Terminator
  Trajectory velocity generation : MATLAB Function  TreatAsAtomicUnit=on
      settings: PermitHierarchicalResolution=ParametersOnly
  UDP receive : Constant  Value=0
  fi_dot : Outport
  robotPose : Outport  Port=2
  desiredVel : Outport  Port=3
  desiredPose : Outport  Port=4
  wires:
  Demux3/2 -> PID Controller4/1
  Rotation Matrix (R(theta))/1(X_w_dot) -> Integrator4/1
  manual/1 -> Switch3/2, Switch2/2
  PID Controller3/1 -> Mux3/1
  Constant/1 -> Switch2/1
  Trajectory velocity generation/1(X_r_dot) -> desiredVel/1, Sum1/1, Integrator1/1
  Sum1/1 -> Inverse Kinematics1/2(u)
  Integrator1/1 -> desiredPose/1, Demux1/1, Scope1/1, Sum2/1
  Mux3/1 -> Sum1/2
  Demux3/3 -> PID Controller5/1
  Demux1/1 -> Terminator3/1
  Forward Kinematics/1(x_dot) -> Rotation Matrix (R(theta))/2(X_R_dot)
  Integrator4/1 -> robotPose/1, Sum2/2, Demux4/1
  t_dep/1 -> Trajectory velocity generation/2(t_dep)
  Inverse Kinematics1/1(fi_dot) -> Scope2/1, Mux/1
  accel/1 -> Trajectory velocity generation/4(accel)
  PID Controller4/1 -> Mux3/2
  Demux4/1 -> Terminator2/1
  Demux4/2 -> Switch3/3
  PID Controller5/1 -> Mux3/3
  Demux3/1 -> PID Controller3/1
  Switch2/1 -> Inverse Kinematics1/1(thetad)
  Switch3/1 -> Rotation Matrix (R(theta))/1(theta)
  Demux1/2 -> Switch2/3
  t/1 -> [t], Trajectory velocity generation/1(t)
  Constant12/1 -> Switch3/1
  Demux/1 -> Forward Kinematics/1(fi_dot)
  Vmax/1 -> Trajectory velocity generation/3(Vmax)
  terminalPose/1 -> Trajectory velocity generation/7(terminalPose)
  omegaMax/1 -> Trajectory velocity generation/5(omegaMax)
  angAccel/1 -> Trajectory velocity generation/6(angAccel)
  departPose/1 -> Trajectory velocity generation/8(departPose)
  Mux/1 -> fi_dot/1
  MATLAB Function1/2(omega) -> Integrator/1, Mux/2
  w_measure/1 -> Demux/1
  resetPose/1 -> Integrator1/2, Integrator4/2
  [t] -> MATLAB Function1/1(t)
  Constant1/1 -> Mux/3
  UDP receive/1 -> Chart/2(kick)
  Integrator/1 -> Chart/3(theta_d)
  Chart/4(departPose) -> MATLAB Function1/5(departPose)
  Chart/1(t_dep) -> MATLAB Function1/2(t_dep)
  Chart/2(omegaMax) -> MATLAB Function1/3(omegaMax)
  Chart/3(terminalPose) -> MATLAB Function1/4(terminalPose)
  MATLAB Function1/1(Ts) -> Display/1
  Sum2/1 -> Scope/1, Demux3/1
  Demux/2 -> Terminator4/1

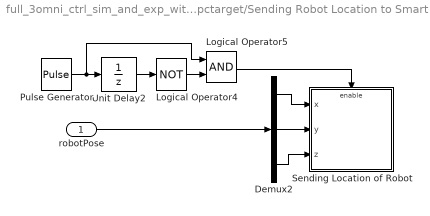
== system full_3omni_ctrl_sim_and_exp_with_xpctarget/Sending Robot Location to Smart Phone ==
  robotPose : Inport
  Demux2 : Demux  Outputs=3
  Logical Operator4 : Logic  Operator=NOT  AllPortsSameDT=off  OutDataTypeStr=boolean
  Logical Operator5 : Logic  AllPortsSameDT=off  OutDataTypeStr=boolean
  Pulse Generator : DiscretePulseGenerator  PulseType=Time based  Period=5  PulseWidth=50
  Sending Location of Robot : Subsystem
  Unit Delay2 : UnitDelay  SampleTime=-1  HasFrameUpgradeWarning=on
  wires:
  Demux2/3 -> Sending Location of Robot/3(z)
  Demux2/2 -> Sending Location of Robot/2(y)
  Demux2/1 -> Sending Location of Robot/1(x)
  Logical Operator5/1 -> Sending Location of Robot/Enable
  robotPose/1 -> Demux2/1
  Pulse Generator/1 -> Logical Operator5/1, Unit Delay2/1
  Unit Delay2/1 -> Logical Operator4/1
  Logical Operator4/1 -> Logical Operator5/2

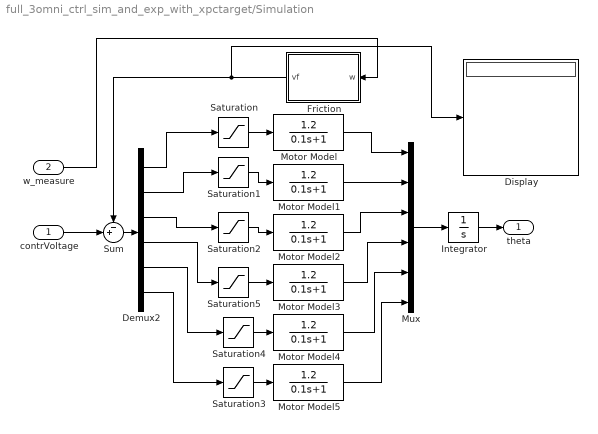
== system full_3omni_ctrl_sim_and_exp_with_xpctarget/Simulation ==
  contrVoltage : Inport
  w_measure : Inport  Port=2
  Demux2 : Demux  Outputs=6
  Display : Display
  Friction : MATLAB Function  TreatAsAtomicUnit=on
      settings: PermitHierarchicalResolution=ParametersOnly
  Integrator : Integrator  InitialCondition=zeros(6,1)
  Motor Model{,1..5} (6 alike) : TransferFcn  Numerator=[1.2]  Denominator=[0.1 1]
  Mux : Mux  Inputs=6
  Saturation{,1..5} (6 alike) : Saturate  UpperLimit=19  LowerLimit=-19
  Sum : Sum  Inputs=-+|
  theta : Outport
  wires:
  contrVoltage/1 -> Sum/2
  Demux2/1 -> Saturation/1
  Motor Model2/1 -> Mux/3
  Motor Model3/1 -> Mux/4
  Motor Model4/1 -> Mux/5
  Motor Model5/1 -> Mux/6
  Demux2/2 -> Saturation1/1
  Demux2/3 -> Saturation2/1
  Demux2/4 -> Saturation5/1
  Demux2/5 -> Saturation4/1
  Demux2/6 -> Saturation3/1
  Mux/1 -> Integrator/1
  Friction/1(vf) -> Display/1, Sum/1
  Sum/1 -> Demux2/1
  w_measure/1 -> Friction/1(w)
  Integrator/1 -> theta/1
  Motor Model/1 -> Mux/1
  Motor Model1/1 -> Mux/2
  Saturation/1 -> Motor Model/1
  Saturation1/1 -> Motor Model1/1
  Saturation2/1 -> Motor Model2/1
  Saturation3/1 -> Motor Model5/1
  Saturation4/1 -> Motor Model4/1
  Saturation5/1 -> Motor Model3/1

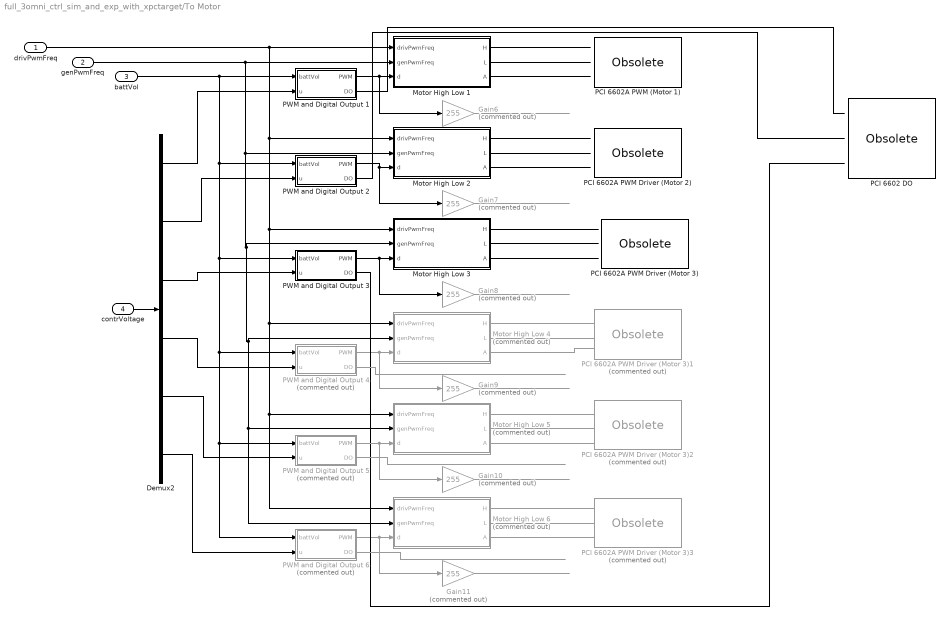
== system full_3omni_ctrl_sim_and_exp_with_xpctarget/To Motor ==
  drivPwmFreq : Inport
  genPwmFreq : Inport  Port=2
  battVol : Inport  Port=3
  contrVoltage : Inport  Port=4
  Demux2 : Demux  Outputs=6
  Gain{6..11} (6 alike) : Gain  Commented=on  Gain=255
  Motor High Low 1 : MATLAB Function  TreatAsAtomicUnit=on
      settings: PermitHierarchicalResolution=ParametersOnly
  Motor High Low 2 : MATLAB Function  TreatAsAtomicUnit=on
      settings: PermitHierarchicalResolution=ParametersOnly
  Motor High Low 3 : MATLAB Function  TreatAsAtomicUnit=on
      settings: PermitHierarchicalResolution=ParametersOnly
  Motor High Low 4 : MATLAB Function  Commented=on  TreatAsAtomicUnit=on
      settings: PermitHierarchicalResolution=ParametersOnly
  Motor High Low 5 : MATLAB Function  Commented=on  TreatAsAtomicUnit=on
      settings: PermitHierarchicalResolution=ParametersOnly
  Motor High Low 6 : MATLAB Function  Commented=on  TreatAsAtomicUnit=on
      settings: PermitHierarchicalResolution=ParametersOnly
  "PCI 6602 DO " : xpcobsoletelib/Obsolete
  PCI 6602A PWM (Motor 1) : xpcobsoletelib/Obsolete
  PCI 6602A PWM Driver (Motor 2) : xpcobsoletelib/Obsolete
  PCI 6602A PWM Driver (Motor 3) : xpcobsoletelib/Obsolete
  PCI 6602A PWM Driver (Motor 3)1 : xpcobsoletelib/Obsolete  Commented=on
  PCI 6602A PWM Driver (Motor 3)2 : xpcobsoletelib/Obsolete  Commented=on
  PCI 6602A PWM Driver (Motor 3)3 : xpcobsoletelib/Obsolete  Commented=on
  PWM and Digital Output 1 : MATLAB Function  TreatAsAtomicUnit=on
      settings: PermitHierarchicalResolution=ParametersOnly
  PWM and Digital Output 2 : MATLAB Function  TreatAsAtomicUnit=on
      settings: PermitHierarchicalResolution=ParametersOnly
  PWM and Digital Output 3 : MATLAB Function  TreatAsAtomicUnit=on
      settings: PermitHierarchicalResolution=ParametersOnly
  PWM and Digital Output 4 : MATLAB Function  Commented=on  TreatAsAtomicUnit=on
      settings: PermitHierarchicalResolution=ParametersOnly
  PWM and Digital Output 5 : MATLAB Function  Commented=on  TreatAsAtomicUnit=on
      settings: PermitHierarchicalResolution=ParametersOnly
  PWM and Digital Output 6 : MATLAB Function  Commented=on  TreatAsAtomicUnit=on
      settings: PermitHierarchicalResolution=ParametersOnly
  wires:
  Motor High Low 6/2(L) -> ?
  PWM and Digital Output 6/1(PWM) -> Gain11/1, Motor High Low 6/3(d)
  drivPwmFreq/1 -> Motor High Low 6/1(drivPwmFreq), Motor High Low 5/1(drivPwmFreq), Motor High Low 4/1(drivPwmFreq), Motor High Low 3/1(drivPwmFreq), Motor High Low 2/1(drivPwmFreq), Motor High Low 1/1(drivPwmFreq)
  Gain11/1 -> ?
  genPwmFreq/1 -> Motor High Low 6/2(genPwmFreq), Motor High Low 5/2(genPwmFreq), Motor High Low 4/2(genPwmFreq), Motor High Low 3/2(genPwmFreq), Motor High Low 2/2(genPwmFreq), Motor High Low 1/2(genPwmFreq)
  Demux2/4 -> PWM and Digital Output 4/2(u)
  Demux2/5 -> PWM and Digital Output 5/2(u)
  PWM and Digital Output 4/1(PWM) -> Gain9/1, Motor High Low 4/3(d)
  Gain9/1 -> ?
  PWM and Digital Output 3/2(DO) -> ?
  battVol/1 -> PWM and Digital Output 2/1(battVol), PWM and Digital Output 3/1(battVol), PWM and Digital Output 4/1(battVol), PWM and Digital Output 5/1(battVol), PWM and Digital Output 6/1(battVol), PWM and Digital Output 1/1(battVol)
  Demux2/2 -> PWM and Digital Output 2/2(u)
  Demux2/3 -> PWM and Digital Output 3/2(u)
  Demux2/6 -> PWM and Digital Output 6/2(u)
  Motor High Low 5/1(H) -> ?
  contrVoltage/1 -> Demux2/1
  Motor High Low 5/3(A) -> ?
  PWM and Digital Output 3/1(PWM) -> Motor High Low 3/3(d), Gain8/1
  PWM and Digital Output 1/1(PWM) -> Motor High Low 1/3(d), Gain6/1
  Motor High Low 6/3(A) -> ?
  Gain10/1 -> ?
  Motor High Low 2/2(L) -> ?
  Gain8/1 -> ?
  Motor High Low 2/3(A) -> ?
  PWM and Digital Output 5/1(PWM) -> Motor High Low 5/3(d), Gain10/1
  Motor High Low 4/1(H) -> ?
  PWM and Digital Output 2/1(PWM) -> Gain7/1, Motor High Low 2/3(d)
  Motor High Low 3/3(A) -> ?
  PWM and Digital Output 2/2(DO) -> ?
  Demux2/1 -> PWM and Digital Output 1/2(u)
  Gain7/1 -> ?
  Motor High Low 3/2(L) -> ?
  PWM and Digital Output 5/2(DO) -> ?
  PWM and Digital Output 4/2(DO) -> ?
  Motor High Low 4/2(L) -> ?
  PWM and Digital Output 6/2(DO) -> ?
  Motor High Low 3/1(H) -> ?
  Motor High Low 4/3(A) -> ?
  PWM and Digital Output 1/2(DO) -> ?
  Gain6/1 -> ?
  Motor High Low 5/2(L) -> ?
  Motor High Low 2/1(H) -> ?
  Motor High Low 6/1(H) -> ?
  Motor High Low 1/3(A) -> ?
  Motor High Low 1/2(L) -> ?
  Motor High Low 1/1(H) -> ?

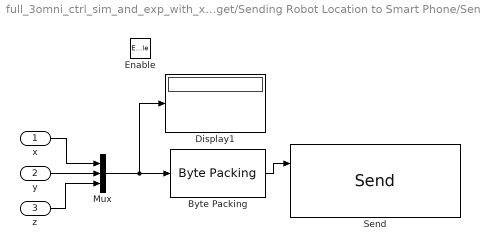
== system full_3omni_ctrl_sim_and_exp_with_xpctarget/Sending Robot Location to Smart Phone/Sending Location of Robot ==
  x : Inport
  y : Inport  Port=2
  z : Inport  Port=3
  Enable : EnablePort
  "Byte Packing " : xpcutilitieslib/Byte Packing   MaskPackedDataType=uint8  MaskUnpackedDataTypes={'double'}  MaskAlignment=1
  Display1 : Display
  Mux : Mux  Inputs=3
  "Send " : slrtlib/UDP/Send   localPort=-1  ipAddress=192.168.88.233  ipPort=2500  sampletime=-1
  wires:
  "Byte Packing "/1 -> "Send "/1
  Mux/1 -> Display1/1, "Byte Packing "/1
  y/1 -> Mux/2
  z/1 -> Mux/3
  x/1 -> Mux/1

== matlab function full_3omni_ctrl_sim_and_exp_with_xpctarget/To Motor/Motor High Low 2 ==
  data: drivPwmFreq input; genPwmFreq input; d input; H output; L output; A output
function [H,L,A]=fcn(drivPwmFreq,genPwmFreq,d)
%genPwmFreq = fm = 80e6;%refrence
%drivPwmFreq = f = 400;%desire
x = genPwmFreq/drivPwmFreq;
H = d*x;
L = (1-d)*x;
A = 1;

== matlab function full_3omni_ctrl_sim_and_exp_with_xpctarget/To Motor/PWM and Digital Output 2 ==
  data: battVol input; u input; PWM output; DO output
function [PWM, DO]= fcn(battVol,u)   %PWM & D(Digital output) are the output and u is the input (Voltage=24V(because DC motor 24V)).
PWM = abs(u)/battVol;               % PWM equals to value of u (voltage value which was applied)
DO = (sign(u)+1)/2;          % (sign(u): included value of u and its sign)so we will get digital ouput between 0 and 1 (if u = 1 => D = 1 or if u = -1 => D =0)

== matlab function full_3omni_ctrl_sim_and_exp_with_xpctarget/To Motor/Motor High Low 3 ==
  data: drivPwmFreq input; genPwmFreq input; d input; H output; L output; A output
function [H,L,A]=fcn(drivPwmFreq,genPwmFreq,d)
%genPwmFreq = fm = 80e6;%refrence
%drivPwmFreq = f = 400;%desire
x = genPwmFreq/drivPwmFreq;
H = d*x;
L = (1-d)*x;
A = 1;

== matlab function full_3omni_ctrl_sim_and_exp_with_xpctarget/To Motor/PWM and Digital Output 3 ==
  data: battVol input; u input; PWM output; DO output
function [PWM, DO]= fcn(battVol,u)   %PWM & D(Digital output) are the output and u is the input (Voltage=24V(because DC motor 24V)).
PWM = abs(u)/battVol;               % PWM equals to value of u (voltage value which was applied)
DO = (sign(u)+1)/2;          % (sign(u): included value of u and its sign)so we will get digital ouput between 0 and 1 (if u = 1 => D = 1 or if u = -1 => D =0)

== matlab function full_3omni_ctrl_sim_and_exp_with_xpctarget/To Motor/Motor High Low 4 ==
  data: drivPwmFreq input; genPwmFreq input; d input; H output; L output; A output
function [H,L,A]=fcn(drivPwmFreq,genPwmFreq,d)
%genPwmFreq = fm = 80e6;%refrence
%drivPwmFreq = f = 400;%desire
x = genPwmFreq/drivPwmFreq;
H = d*x;
L = (1-d)*x;
A = 1;

== matlab function full_3omni_ctrl_sim_and_exp_with_xpctarget/To Motor/PWM and Digital Output 4 ==
  data: battVol input; u input; PWM output; DO output
function [PWM, DO]= fcn(battVol,u)   %PWM & D(Digital output) are the output and u is the input (Voltage=24V(because DC motor 24V)).
PWM = abs(u)/battVol;               % PWM equals to value of u (voltage value which was applied)
DO = (sign(u)+1)/2;          % (sign(u): included value of u and its sign)so we will get digital ouput between 0 and 1 (if u = 1 => D = 1 or if u = -1 => D =0)

== matlab function full_3omni_ctrl_sim_and_exp_with_xpctarget/To Motor/Motor High Low 5 ==
  data: drivPwmFreq input; genPwmFreq input; d input; H output; L output; A output
function [H,L,A]=fcn(drivPwmFreq,genPwmFreq,d)
%genPwmFreq = fm = 80e6;%refrence
%drivPwmFreq = f = 400;%desire
x = genPwmFreq/drivPwmFreq;
H = d*x;
L = (1-d)*x;
A = 1;

== matlab function full_3omni_ctrl_sim_and_exp_with_xpctarget/To Motor/PWM and Digital Output 1 ==
  data: battVol input; u input; PWM output; DO output
function [PWM, DO]= fcn(battVol,u)   %PWM & D(Digital output) are the output and u is the input (Voltage=24V(because DC motor 24V)).
PWM = abs(u)/battVol;               % PWM equals to value of u (voltage value which was applied)
DO = (sign(u)+1)/2;          % (sign(u): included value of u and its sign)so we will get digital ouput between 0 and 1 (if u = 1 => D = 1 or if u = -1 => D =0)

== matlab function full_3omni_ctrl_sim_and_exp_with_xpctarget/To Motor/Motor High Low 1 ==
  data: drivPwmFreq input; genPwmFreq input; d input; H output; L output; A output
function [H,L,A]=fcn(drivPwmFreq,genPwmFreq,d)
%genPwmFreq = fm = 80e6;%refrence
%drivPwmFreq = f = 400;%desire
x = genPwmFreq/drivPwmFreq;
H = d*x;
L = (1-d)*x;
A = 1;

== matlab function full_3omni_ctrl_sim_and_exp_with_xpctarget/To Motor/PWM and Digital Output 5 ==
  data: battVol input; u input; PWM output; DO output
function [PWM, DO]= fcn(battVol,u)   %PWM & D(Digital output) are the output and u is the input (Voltage=24V(because DC motor 24V)).
PWM = abs(u)/battVol;               % PWM equals to value of u (voltage value which was applied)
DO = (sign(u)+1)/2;          % (sign(u): included value of u and its sign)so we will get digital ouput between 0 and 1 (if u = 1 => D = 1 or if u = -1 => D =0)

== matlab function full_3omni_ctrl_sim_and_exp_with_xpctarget/To Motor/Motor High Low 6 ==
  data: drivPwmFreq input; genPwmFreq input; d input; H output; L output; A output
function [H,L,A]=fcn(drivPwmFreq,genPwmFreq,d)
%genPwmFreq = fm = 80e6;%refrence
%drivPwmFreq = f = 400;%desire
x = genPwmFreq/drivPwmFreq;
H = d*x;
L = (1-d)*x;
A = 1;

== matlab function full_3omni_ctrl_sim_and_exp_with_xpctarget/To Motor/PWM and Digital Output 6 ==
  data: battVol input; u input; PWM output; DO output
function [PWM, DO]= fcn(battVol,u)   %PWM & D(Digital output) are the output and u is the input (Voltage=24V(because DC motor 24V)).
PWM = abs(u)/battVol;               % PWM equals to value of u (voltage value which was applied)
DO = (sign(u)+1)/2;          % (sign(u): included value of u and its sign)so we will get digital ouput between 0 and 1 (if u = 1 => D = 1 or if u = -1 => D =0)

== matlab function full_3omni_ctrl_sim_and_exp_with_xpctarget/From Encoder/Convert pulse to rad1 ==
  data: u input; ppr input; gearRatio input; outGearBox output
function outGearBox = fcn(u,ppr,gearRatio)

persistent counter_num over_flag
if(isempty(counter_num)), counter_num = 0;end
if(isempty(over_flag)), over_flag = 0;end
pulse2radian = 2*pi/ppr; % 1 pulse = ?? radian

if(double(u) - counter_num > 40000), over_flag = over_flag-1;
elseif(double(u) - counter_num < -40000), over_flag = over_flag+1;
end

inGearBox = (double(u)+over_flag*(2^32 -1))*pulse2radian; 
outGearBox = inGearBox/gearRatio;
counter_num = double(u) ;

== matlab function full_3omni_ctrl_sim_and_exp_with_xpctarget/From Encoder/Convert pulse to rad2 ==
  data: u input; ppr input; gearRatio input; outGearBox output
function outGearBox = fcn(u,ppr,gearRatio)

persistent counter_num over_flag
if(isempty(counter_num)), counter_num = 0;end
if(isempty(over_flag)), over_flag = 0;end
pulse2radian = 2*pi/ppr; % 1 pulse = ?? radian

if(double(u) - counter_num > 40000), over_flag = over_flag-1;
elseif(double(u) - counter_num < -40000), over_flag = over_flag+1;
end

inGearBox = (double(u)+over_flag*(2^32 -1))*pulse2radian; 
outGearBox = inGearBox/gearRatio;
counter_num = double(u) ;

== matlab function full_3omni_ctrl_sim_and_exp_with_xpctarget/From Encoder/Convert pulse to rad3 ==
  data: u input; ppr input; gearRatio input; outGearBox output
function outGearBox = fcn(u,ppr,gearRatio)

persistent counter_num over_flag
if(isempty(counter_num)), counter_num = 0;end
if(isempty(over_flag)), over_flag = 0;end
pulse2radian = 2*pi/ppr; % 1 pulse = ?? radian

if(double(u) - counter_num > 40000), over_flag = over_flag-1;
elseif(double(u) - counter_num < -40000), over_flag = over_flag+1;
end

inGearBox = (double(u)+over_flag*(2^32 -1))*pulse2radian; 
outGearBox = inGearBox/gearRatio;
counter_num = double(u) ;

== matlab function full_3omni_ctrl_sim_and_exp_with_xpctarget/From Encoder/Convert pulse to rad4 ==
  data: u input; ppr input; gearRatio input; outGearBox output
function outGearBox = fcn(u,ppr,gearRatio)

persistent counter_num over_flag
if(isempty(counter_num)), counter_num = 0;end
if(isempty(over_flag)), over_flag = 0;end
pulse2radian = 2*pi/ppr; % 1 pulse = ?? radian

if(double(u) - counter_num > 40000), over_flag = over_flag-1;
elseif(double(u) - counter_num < -40000), over_flag = over_flag+1;
end

inGearBox = (double(u)+over_flag*(2^32 -1))*pulse2radian; 
outGearBox = inGearBox/gearRatio;
counter_num = double(u) ;

== matlab function full_3omni_ctrl_sim_and_exp_with_xpctarget/From Encoder/Convert pulse to rad5 ==
  data: u input; ppr input; gearRatio input; outGearBox output
function outGearBox = fcn(u,ppr,gearRatio)

persistent counter_num over_flag
if(isempty(counter_num)), counter_num = 0;end
if(isempty(over_flag)), over_flag = 0;end
pulse2radian = 2*pi/ppr; % 1 pulse = ?? radian

if(double(u) - counter_num > 40000), over_flag = over_flag-1;
elseif(double(u) - counter_num < -40000), over_flag = over_flag+1;
end

inGearBox = (double(u)+over_flag*(2^32 -1))*pulse2radian; 
outGearBox = inGearBox/gearRatio;
counter_num = double(u) ;

== matlab function full_3omni_ctrl_sim_and_exp_with_xpctarget/From Encoder/Convert pulse to rad6 ==
  data: u input; ppr input; gearRatio input; outGearBox output
function outGearBox = fcn(u,ppr,gearRatio)

persistent counter_num over_flag
if(isempty(counter_num)), counter_num = 0;end
if(isempty(over_flag)), over_flag = 0;end
pulse2radian = 2*pi/ppr; % 1 pulse = ?? radian

if(double(u) - counter_num > 40000), over_flag = over_flag-1;
elseif(double(u) - counter_num < -40000), over_flag = over_flag+1;
end

inGearBox = (double(u)+over_flag*(2^32 -1))*pulse2radian; 
outGearBox = inGearBox/gearRatio;
counter_num = double(u) ;
